simulink subsystem "s2EM"  (R2023b)
settings: Solver=VariableStepAuto  StartTime=0.0  StopTime=10.0  RelTol=1e-3
settings Model: Creator=The MathWorks, Inc.  LastModifiedBy=The MathWorks, Inc.

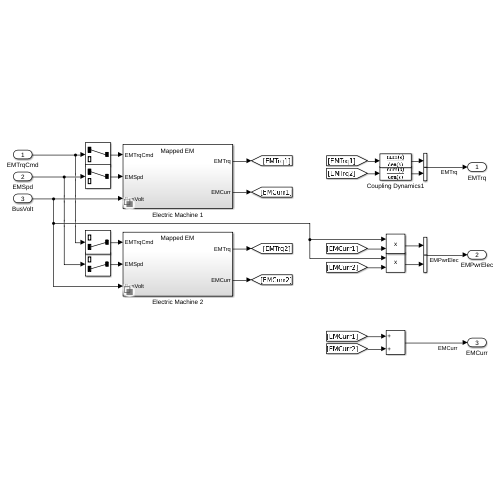
[thumbnail: Simulink's stored preview of the top-level diagram]
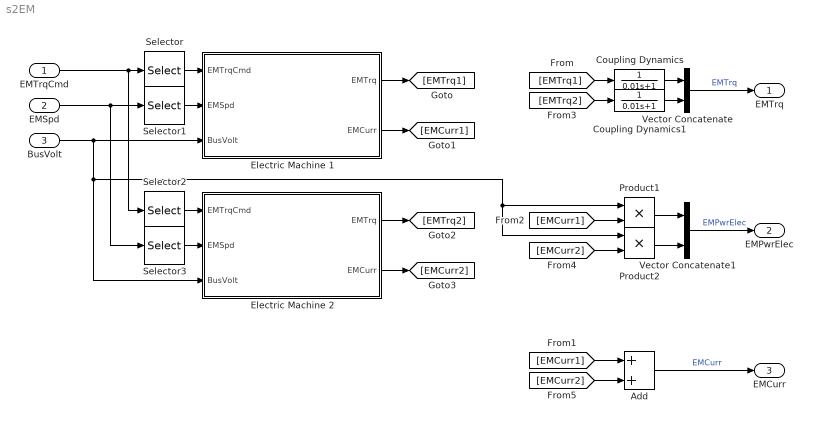
== system s2EM ==
  EMTrqCmd : Inport
  EMSpd : Inport  Port=2
  BusVolt : Inport  Port=3
  Add : Sum
  Coupling Dynamics : TransferFcn  Denominator=[0.01 1]
  Coupling Dynamics1 : TransferFcn  Denominator=[0.01 1]
  Electric Machine 1 : Subsystem  Variant=on  VariantControlMode=label  LabelModeActiveChoice=Mapped EM
  Electric Machine 2 : Subsystem  Variant=on  VariantControlMode=label  LabelModeActiveChoice=Mapped EM
  Product1 : Product
  Product2 : Product
  Selector : Selector  InputPortWidth=2  IndexOptions=Index vector (dialog)  Indices=[1]  OutputSizes=1
  Selector1 : Selector  InputPortWidth=2  IndexOptions=Index vector (dialog)  Indices=[1]  OutputSizes=1
  Selector2 : Selector  InputPortWidth=2  IndexOptions=Index vector (dialog)  Indices=[2]  OutputSizes=1
  Selector3 : Selector  InputPortWidth=2  IndexOptions=Index vector (dialog)  Indices=[2]  OutputSizes=1
  Vector Concatenate : Concatenate
  Vector Concatenate1 : Concatenate
  EMTrq : Outport
  EMPwrElec : Outport  Port=2
  EMCurr : Outport  Port=3
  wires:
  Electric Machine 2/2(EMCurr) -> [EMCurr2]
  Electric Machine 2/1(EMTrq) -> [EMTrq2]
  [EMCurr2] -> Add/2
  [EMCurr2] -> Product2/2
  [EMTrq2] -> Coupling Dynamics1/1
  [EMCurr1] -> Product1/2
  [EMCurr1] -> Add/1
  Electric Machine 1/2(EMCurr) -> [EMCurr1]
  [EMTrq1] -> Coupling Dynamics/1
  Electric Machine 1/1(EMTrq) -> [EMTrq1]
  EMSpd/1 -> Selector1/1, Selector3/1
  Selector/1 -> Electric Machine 1/1(EMTrqCmd)
  Add/1 -> EMCurr/1  "EMCurr"
  Selector2/1 -> Electric Machine 2/1(EMTrqCmd)
  Coupling Dynamics1/1 -> Vector Concatenate/2
  Product2/1 -> Vector Concatenate1/2
  Product1/1 -> Vector Concatenate1/1
  EMTrqCmd/1 -> Selector/1, Selector2/1
  Selector3/1 -> Electric Machine 2/2(EMSpd)
  Selector1/1 -> Electric Machine 1/2(EMSpd)
  Vector Concatenate1/1 -> EMPwrElec/1  "EMPwrElec"
  Coupling Dynamics/1 -> Vector Concatenate/1
  BusVolt/1 -> Product2/1, Product1/1, Electric Machine 2/3(BusVolt), Electric Machine 1/3(BusVolt)
  Vector Concatenate/1 -> EMTrq/1  "EMTrq"

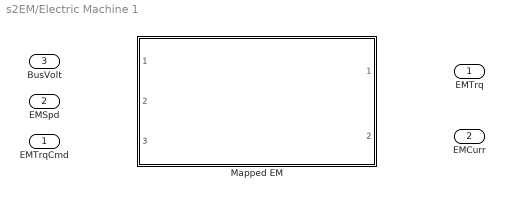
== system s2EM/Electric Machine 1 ==
  EMTrqCmd : Inport
  EMSpd : Inport  Port=2
  BusVolt : Inport  Port=3
  Mapped EM : Subsystem  VariantControl=Mapped EM  ReferencedSubsystem=ElectricMachine1
  EMTrq : Outport  VectorParamsAs1DForOutWhenUnconnected=off
  EMCurr : Outport  Port=2  VectorParamsAs1DForOutWhenUnconnected=off

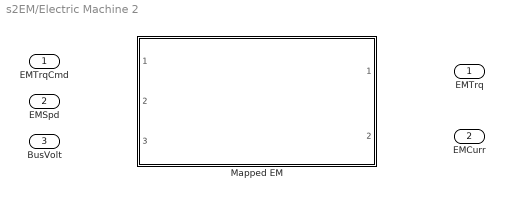
== system s2EM/Electric Machine 2 ==
  EMTrqCmd : Inport
  EMSpd : Inport  Port=2
  BusVolt : Inport  Port=3
  Mapped EM : Subsystem  VariantControl=Mapped EM  ReferencedSubsystem=ElectricMachine2
  EMTrq : Outport  VectorParamsAs1DForOutWhenUnconnected=off
  EMCurr : Outport  Port=2  VectorParamsAs1DForOutWhenUnconnected=off
